simulink library "Enrg_conv_El_to_Mec_zfCetrax"  (R2016a)
settings: Solver=ode1  StartTime=0.0  StopTime=Inf  FixedStep=0.001  RelTol=1e-3
undefined symbols (not defined in the file): drvEmot_RefTqeMOT, FirstDrivenAxle_FirstDrivenAxleNoOfEmot, FirstDrivenAxleNoOfEmot, FMIKit, mec_fRollCoeffOverall, mec_iDiffAxle, mec_massVehicle_kg, mec_rWheelDriven, RefTqeMOT, SecondDrivenAxle_SecondDrivenAxleNoOfEmot, SecondDrivenAxleNoOfEmot
libraries: simulink_extras x3, Enrg_conv_El_to_Mec_zfCetrax x3
(part 2 of 3)

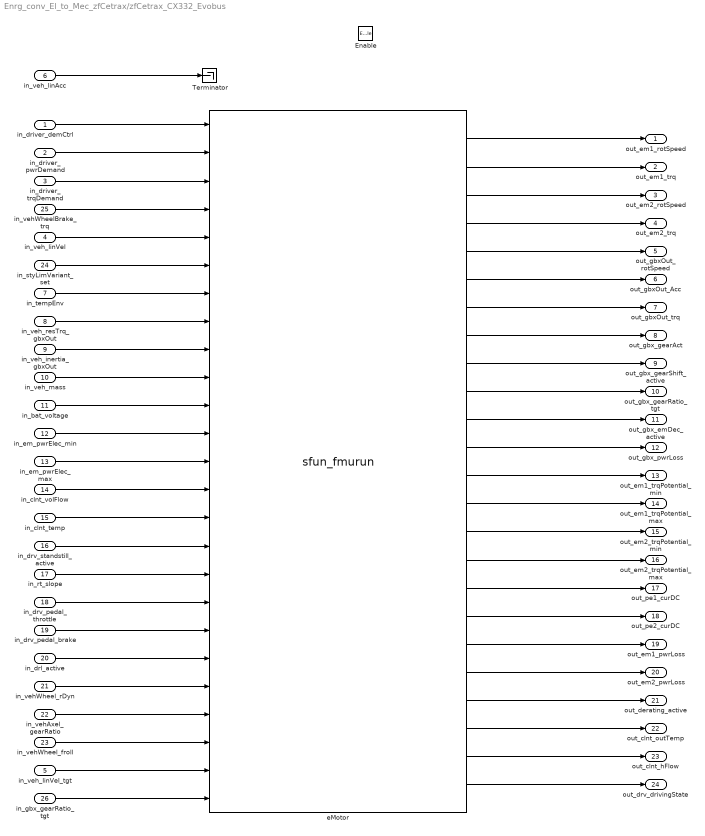
== system Enrg_conv_El_to_Mec_zfCetrax/zfCetrax_CX332_Evobus ==
  in_driver_demCtrl : Inport
  in_driver_pwrDemand : Inport  Port=2
  in_driver_trqDemand : Inport  Port=3
  in_veh_linVel : Inport  Port=4
  in_veh_linVel_tgt : Inport  Port=5
  in_veh_linAcc : Inport  Port=6
  in_tempEnv : Inport  Port=7
  in_veh_resTrq_gbxOut : Inport  Port=8
  in_veh_inertia_gbxOut : Inport  Port=9
  in_veh_mass : Inport  Port=10
  in_bat_voltage : Inport  Port=11
  in_em_pwrElec_min : Inport  Port=12
  in_em_pwrElec_max : Inport  Port=13
  in_clnt_volFlow : Inport  Port=14
  in_clnt_temp : Inport  Port=15
  in_drv_standstill_active : Inport  Port=16
  in_rt_slope : Inport  Port=17
  in_drv_pedal_throttle : Inport  Port=18
  in_drv_pedal_brake : Inport  Port=19
  in_drl_active : Inport  Port=20
  in_vehWheel_rDyn : Inport  Port=21
  in_vehAxel_gearRatio : Inport  Port=22
  in_vehWheel_froll : Inport  Port=23
  in_styLimVariant_set : Inport  Port=24
  in_vehWheelBrake_trq : Inport  Port=25
  in_gbx_gearRatio_tgt : Inport  Port=26
  Enable : EnablePort
  Terminator : Terminator
  eMotor : S-Function  LoadFcn=FMIKit.setSFunctionParameters(gcb)  FunctionName=sfun_fmurun  Parameters='2.0' 1 '{72cfe2f2-dd7d-8c89-a52c-23a74381eb1f}' 'CustomerVar_EvoBusCX332' FMIKit.getUnzipDirectory(gcb) 0 0 0 '' 0 -1 0 0 0 [] [] [] [] char({}) [1 1 1 1 1 1 1 1 1 1 1 1 1 1 1 1 1 1 1 1 1 1 1 1 1] [0 0 0 0 0 0 0 0 0 0 0 0 0 0 0 0 0 0 0 0 0 0 0 0 0] [0 0 0 0 0 0 0 0 0 0 0 0 0 0 0 0 0 0 0 0 0 0 0 0 0] [0 1 2 3 4 5 6 7 8 9 10 11 12 13 14 15 16 17 18 19 20 21 22 23 24] [1 1 1 1 1 1 1 1 1 1 1 1 1 1 1 1 1 1 1 1 1 1 1 1] [0 0 0 0 0 0 0 0 0 0 0 0 0 0 0 0 0 0 0 0 0 0 0 0] [25 26 27 28 29 30 31 32 33 34 35 36 37 38 39 40 41 42 43 44 45 46 47 48]  SFunctionDeploymentMode=off  EnableBusSupport=off
      settings: DeleteFcn=FMIKit.closeBlockDialog(gcbh)  ModelCloseFcn=FMIKit.closeBlockDialog(gcbh)  DestroyFcn=FMIKit.closeBlockDialog(gcbh)  OpenFcn=FMIKit.showBlockDialog(gcbh);  CloseFcn=FMIKit.closeBlockDialog(gcbh)  ParentCloseFcn=FMIKit.closeBlockDialog(gcbh)
      mask Help: eval('FMIKit.showBlockDialogHelp();')
      mask Display:
      | ports = get_param(gcb, 'Ports');
      | 
      | inports = FMIKit.getInportLabels(gcb);
      | 
      | for i = 1:min(numel(inports), ports(1))
      |     port_label('input', i, inports{i})
      | end
      | 
      | outports = FMIKit.getOutportLabels(gcb);
      | 
      | for i = 1:min(numel(outports), ports(2))
      |     port_label('output', i, outports{i})
      | end
      | 
      | if isempty(inports) && isempty(outports)
      |     patch([-20 65, 65 -20], [-20 -20 70 70], [1 1 1])
      |     plot([-2 50 50 -2 -2], [0 0 50 50 0])
      |     patch([-9 12 12 -9 -9], [12 12 20 20 12], [1 1 1])
      |     plot([-9 12 12 -9 -9], [12 12 20 20 12])
      |     patch([-9 12 12 -9 -9], [30 30 38 38 30], [1 1 1])
      |     plot([-9 12 12 -9 -9], [30 30 38 38 30])
      | end
  out_em1_rotSpeed : Outport
  out_em1_trq : Outport  Port=2
  out_em2_rotSpeed : Outport  Port=3
  out_em2_trq : Outport  Port=4
  out_gbxOut_rotSpeed : Outport  Port=5
  out_gbxOut_Acc : Outport  Port=6
  out_gbxOut_trq : Outport  Port=7
  out_gbx_gearAct : Outport  Port=8
  out_gbx_gearShift_active : Outport  Port=9
  out_gbx_gearRatio_tgt : Outport  Port=10
  out_gbx_emDec_active : Outport  Port=11
  out_gbx_pwrLoss : Outport  Port=12
  out_em1_trqPotential_min : Outport  Port=13
  out_em1_trqPotential_max : Outport  Port=14
  out_em2_trqPotential_min : Outport  Port=15
  out_em2_trqPotential_max : Outport  Port=16
  out_pe1_curDC : Outport  Port=17
  out_pe2_curDC : Outport  Port=18
  out_em1_pwrLoss : Outport  Port=19
  out_em2_pwrLoss : Outport  Port=20
  out_derating_active : Outport  Port=21
  out_clnt_outTemp : Outport  Port=22
  out_clnt_hFlow : Outport  Port=23
  out_drv_drivingState : Outport  Port=24
  wires:
  eMotor/24 -> out_drv_drivingState/1
  in_gbx_gearRatio_tgt/1 -> eMotor/25
  in_vehWheel_froll/1 -> eMotor/23
  in_vehAxel_gearRatio/1 -> eMotor/22
  in_vehWheel_rDyn/1 -> eMotor/21
  in_driver_demCtrl/1 -> eMotor/1
  in_driver_trqDemand/1 -> eMotor/3
  in_veh_linVel/1 -> eMotor/5
  in_veh_linVel_tgt/1 -> eMotor/24
  in_tempEnv/1 -> eMotor/7
  in_veh_resTrq_gbxOut/1 -> eMotor/8
  in_veh_inertia_gbxOut/1 -> eMotor/9
  in_veh_mass/1 -> eMotor/10
  in_bat_voltage/1 -> eMotor/11
  in_em_pwrElec_min/1 -> eMotor/12
  in_em_pwrElec_max/1 -> eMotor/13
  in_clnt_volFlow/1 -> eMotor/14
  in_clnt_temp/1 -> eMotor/15
  in_drv_standstill_active/1 -> eMotor/16
  in_rt_slope/1 -> eMotor/17
  in_drv_pedal_throttle/1 -> eMotor/18
  in_drv_pedal_brake/1 -> eMotor/19
  in_drl_active/1 -> eMotor/20
  in_driver_pwrDemand/1 -> eMotor/2
  in_veh_linAcc/1 -> Terminator/1
  eMotor/1 -> out_em1_rotSpeed/1
  eMotor/2 -> out_em1_trq/1
  eMotor/3 -> out_em2_rotSpeed/1
  eMotor/4 -> out_em2_trq/1
  eMotor/5 -> out_gbxOut_rotSpeed/1
  eMotor/6 -> out_gbxOut_Acc/1
  eMotor/7 -> out_gbxOut_trq/1
  eMotor/8 -> out_gbx_gearAct/1
  eMotor/9 -> out_gbx_gearShift_active/1
  eMotor/10 -> out_gbx_gearRatio_tgt/1
  eMotor/11 -> out_gbx_emDec_active/1
  eMotor/12 -> out_gbx_pwrLoss/1
  eMotor/13 -> out_em1_trqPotential_min/1
  eMotor/14 -> out_em1_trqPotential_max/1
  eMotor/15 -> out_em2_trqPotential_min/1
  eMotor/16 -> out_em2_trqPotential_max/1
  eMotor/17 -> out_pe1_curDC/1
  eMotor/18 -> out_pe2_curDC/1
  eMotor/19 -> out_em1_pwrLoss/1
  eMotor/20 -> out_em2_pwrLoss/1
  eMotor/21 -> out_derating_active/1
  eMotor/22 -> out_clnt_outTemp/1
  eMotor/23 -> out_clnt_hFlow/1
  in_styLimVariant_set/1 -> eMotor/6
  in_vehWheelBrake_trq/1 -> eMotor/4

== system Enrg_conv_El_to_Mec_zfCetrax/EDB_DriveEmot_zfCetrax/EMD1_Selection ==
  pti_EMD1_TrqReq_Nm : Inport
  pti_EMD1_ControlMode : Inport  Port=2
  edcu_EMD1_CMD_TorqueRefLim : Inport  Port=3
  edcu_EMD1_CMD_ControlMode : Inport  Port=4
  Bus Creator1 : BusCreator  Inputs=2
  Bus Creator2 : BusCreator  Inputs=2
  Constant2 : Constant  Value=0
  Constant3 : Constant  Value=-1
  Constant4 : Constant  Value=drvEmot_RefTqeMOT
  Logical Operator : Logic  Operator=NOT  AllPortsSameDT=off  OutDataTypeStr=boolean
  Logical Operator1 : Logic  AllPortsSameDT=off  OutDataTypeStr=boolean
  Relational Operator2 : RelationalOperator  Operator===  OutDataTypeStr=boolean
  Relational Operator3 : RelationalOperator  Operator===  OutDataTypeStr=boolean
  Switch : Switch  Criteria=u2 > Threshold
  percent_to_Nm2 : Subsystem
  Signal : Outport
  wires:
  Constant2/1 -> Relational Operator2/2
  Relational Operator2/1 -> Logical Operator1/1
  Constant3/1 -> Relational Operator3/1
  Relational Operator3/1 -> Logical Operator1/2
  edcu_EMD1_CMD_ControlMode/1 -> Bus Creator2/2  "EMD1_ControlMode"
  Switch/1 -> Signal/1
  edcu_EMD1_CMD_TorqueRefLim/1 -> percent_to_Nm2/1(Percentage_Torque)
  Bus Creator2/1 -> Switch/3
  pti_EMD1_ControlMode/1 -> Bus Creator1/2, Relational Operator3/2  "EMD1_ControlMode"
  pti_EMD1_TrqReq_Nm/1 -> Relational Operator2/1, Bus Creator1/1  "EMD1_TrqReq_Nm"
  Constant4/1 -> percent_to_Nm2/2(Reference_Torque)
  percent_to_Nm2/1(Torque_Nm) -> Bus Creator2/1  "EMD1_TrqReq_Nm"
  Logical Operator1/1 -> Logical Operator/1
  Bus Creator1/1 -> Switch/1
  Logical Operator/1 -> Switch/2

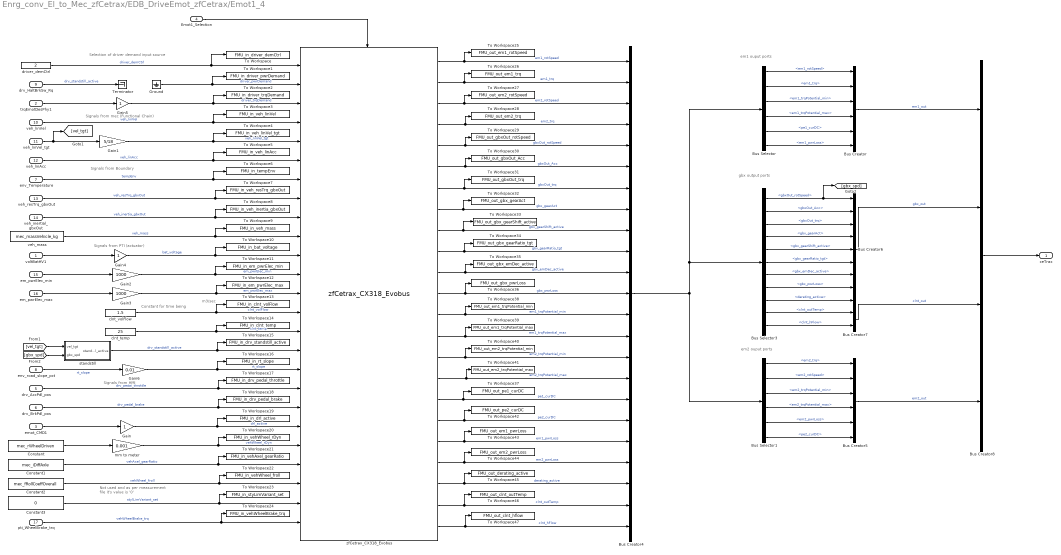
== system Enrg_conv_El_to_Mec_zfCetrax/EDB_DriveEmot_zfCetrax/Emot1_4 ==
  note: em1 ouput ports
  note: Selection of driver demand input source
  note: Signals from Boundary
  note: Signals from HMI
  note: Signals from mec (Functional Chain)
  note: Constant for time being
  note: Signals from PTI (actuator)
  note: em2 ouput ports
  note: gbx output ports
  note: Not used and as per
      | measurement file it's value is '0'
  note: m3/sec
  voltBatHV1 : Inport
  trqEmotDesPhy1 : Inport  Port=2
  emot_CMD1 : Inport  Port=3
  Emot1_Selection : Inport  Port=4
  drv_AccPdl_pos : Inport  Port=5
  drv_BrkPdl_pos : Inport  Port=6
  env_Temperature : Inport  Port=7
  env_road_slope_pct : Inport  Port=8
  drv_HaltBrkSw_Rq : Inport  Port=9
  veh_linVel : Inport  Port=10
  veh_linVel_tgt : Inport  Port=11
  veh_linAcc : Inport  Port=12
  veh_resTrq_gbxOut : Inport  Port=13
  veh_inertial_gbxOut : Inport  Port=14
  em_pwrElec_min : Inport  Port=15
  em_pwrElec_max : Inport  Port=16
  pti_WheelBrake_trq : Inport  Port=17
  Bus Creator : BusCreator  Inputs=6
  Bus Creator4 : BusCreator  Inputs=23
  Bus Creator5 : BusCreator  Inputs=6
  Bus Creator6 : BusCreator  Inputs=9
  Bus Creator7 : BusCreator  Inputs=2
  Bus Creator8 : BusCreator  Inputs=4
  Bus Selector : BusSelector  OutputSignals=em1_rotSpeed,em1_trq,em1_trqPotential_min,em1_trqPotential_max,pe1_curDC,em1_pwrLoss
  Bus Selector1 : BusSelector  OutputSignals=em2_trq,em2_rotSpeed,em2_trqPotential_min,em2_trqPotential_max,em2_pwrLoss,pe2_curDC
  Bus Selector3 : BusSelector  OutputSignals=gbxOut_rotSpeed,gbxOut_Acc,gbxOut_trq,gbx_gearAct,gbx_gearShift_active,gbx_gearRatio_tgt,gbx_emDec_active,gbx_pwrLoss,derating_active,clnt_outTemp,clnt_hFlow
  Constant : Constant  Value=mec_rWheelDriven
  Constant1 : Constant  Value=mec_iDiffAxle
  Constant2 : Constant  Value=mec_fRollCoeffOverall
  Constant3 : Constant  Value=0
  Gain : Gain
  Gain1 : Gain  Gain=5/18
  Gain2 : Gain  Gain=1000
  Gain3 : Gain  Gain=1000
  Gain4 : Gain
  Gain5 : Gain
  Gain6 : Gain  Gain=0.01
  Ground : Ground
  Terminator : Terminator
  To Workspace : ToWorkspace  VariableName=FMU_in_driver_demCtrl  SampleTime=-1
      settings: Save2DSignal=2-D array (concatenate along first dimension)
  To Workspace1 : ToWorkspace  VariableName=FMU_in_driver_pwrDemand  SampleTime=-1
      settings: Save2DSignal=2-D array (concatenate along first dimension)
  To Workspace10 : ToWorkspace  VariableName=FMU_in_bat_voltage  SampleTime=-1
      settings: Save2DSignal=2-D array (concatenate along first dimension)
  To Workspace11 : ToWorkspace  VariableName=FMU_in_em_pwrElec_min  SampleTime=-1
      settings: Save2DSignal=2-D array (concatenate along first dimension)
  To Workspace12 : ToWorkspace  VariableName=FMU_in_em_pwrElec_max  SampleTime=-1
      settings: Save2DSignal=2-D array (concatenate along first dimension)
  To Workspace13 : ToWorkspace  VariableName=FMU_in_clnt_volFlow  SampleTime=-1
      settings: Save2DSignal=2-D array (concatenate along first dimension)
  To Workspace14 : ToWorkspace  VariableName=FMU_in_clnt_temp  SampleTime=-1
      settings: Save2DSignal=2-D array (concatenate along first dimension)
  To Workspace15 : ToWorkspace  VariableName=FMU_in_drv_standstill_active  SampleTime=-1
      settings: Save2DSignal=2-D array (concatenate along first dimension)
  To Workspace16 : ToWorkspace  VariableName=FMU_in_rt_slope  SampleTime=-1
      settings: Save2DSignal=2-D array (concatenate along first dimension)
  To Workspace17 : ToWorkspace  VariableName=FMU_in_drv_pedal_throttle  SampleTime=-1
      settings: Save2DSignal=2-D array (concatenate along first dimension)
  To Workspace18 : ToWorkspace  VariableName=FMU_in_drv_pedal_brake  SampleTime=-1
      settings: Save2DSignal=2-D array (concatenate along first dimension)
  To Workspace19 : ToWorkspace  VariableName=FMU_in_drl_active  SampleTime=-1
      settings: Save2DSignal=2-D array (concatenate along first dimension)
  To Workspace2 : ToWorkspace  VariableName=FMU_in_driver_trqDemand  SampleTime=-1
      settings: Save2DSignal=2-D array (concatenate along first dimension)
  To Workspace20 : ToWorkspace  VariableName=FMU_in_vehWheel_rDyn  SampleTime=-1
      settings: Save2DSignal=2-D array (concatenate along first dimension)
  To Workspace21 : ToWorkspace  VariableName=FMU_in_vehAxel_gearRatio  SampleTime=-1
      settings: Save2DSignal=2-D array (concatenate along first dimension)
  To Workspace22 : ToWorkspace  VariableName=FMU_in_vehWheel_froll  SampleTime=-1
      settings: Save2DSignal=2-D array (concatenate along first dimension)
  To Workspace23 : ToWorkspace  VariableName=FMU_in_styLimVariant_set  SampleTime=-1
      settings: Save2DSignal=2-D array (concatenate along first dimension)
  To Workspace24 : ToWorkspace  VariableName=FMU_in_vehWheelBrake_trq  SampleTime=-1
      settings: Save2DSignal=2-D array (concatenate along first dimension)
  To Workspace25 : ToWorkspace  VariableName=FMU_out_em1_rotSpeed  SampleTime=-1
      settings: Save2DSignal=2-D array (concatenate along first dimension)
  To Workspace26 : ToWorkspace  VariableName=FMU_out_em1_trq  SampleTime=-1
      settings: Save2DSignal=2-D array (concatenate along first dimension)
  To Workspace27 : ToWorkspace  VariableName=FMU_out_em2_rotSpeed  SampleTime=-1
      settings: Save2DSignal=2-D array (concatenate along first dimension)
  To Workspace28 : ToWorkspace  VariableName=FMU_out_em2_trq  SampleTime=-1
      settings: Save2DSignal=2-D array (concatenate along first dimension)
  To Workspace29 : ToWorkspace  VariableName=FMU_out_gbxOut_rotSpeed  SampleTime=-1
      settings: Save2DSignal=2-D array (concatenate along first dimension)
  To Workspace3 : ToWorkspace  VariableName=FMU_in_veh_linVel  SampleTime=-1
      settings: Save2DSignal=2-D array (concatenate along first dimension)
  To Workspace30 : ToWorkspace  VariableName=FMU_out_gbxOut_Acc  SampleTime=-1
      settings: Save2DSignal=2-D array (concatenate along first dimension)
  To Workspace31 : ToWorkspace  VariableName=FMU_out_gbxOut_trq  SampleTime=-1
      settings: Save2DSignal=2-D array (concatenate along first dimension)
  To Workspace32 : ToWorkspace  VariableName=FMU_out_gbx_gearAct  SampleTime=-1
      settings: Save2DSignal=2-D array (concatenate along first dimension)
  To Workspace33 : ToWorkspace  VariableName=FMU_out_gbx_gearShift_active  SampleTime=-1
      settings: Save2DSignal=2-D array (concatenate along first dimension)
  To Workspace34 : ToWorkspace  VariableName=FMU_out_gbx_gearRatio_tgt  SampleTime=-1
      settings: Save2DSignal=2-D array (concatenate along first dimension)
  To Workspace35 : ToWorkspace  VariableName=FMU_out_gbx_emDec_active  SampleTime=-1
      settings: Save2DSignal=2-D array (concatenate along first dimension)
  To Workspace36 : ToWorkspace  VariableName=FMU_out_gbx_pwrLoss  SampleTime=-1
      settings: Save2DSignal=2-D array (concatenate along first dimension)
  To Workspace37 : ToWorkspace  VariableName=FMU_out_pe1_curDC  SampleTime=-1
      settings: Save2DSignal=2-D array (concatenate along first dimension)
  To Workspace38 : ToWorkspace  VariableName=FMU_out_em1_trqPotential_min  SampleTime=-1
      settings: Save2DSignal=2-D array (concatenate along first dimension)
  To Workspace39 : ToWorkspace  VariableName=FMU_out_em1_trqPotential_max  SampleTime=-1
      settings: Save2DSignal=2-D array (concatenate along first dimension)
  To Workspace4 : ToWorkspace  VariableName=FMU_in_veh_linVel_tgt  SampleTime=-1
      settings: Save2DSignal=2-D array (concatenate along first dimension)
  To Workspace40 : ToWorkspace  VariableName=FMU_out_em2_trqPotential_min  SampleTime=-1
      settings: Save2DSignal=2-D array (concatenate along first dimension)
  To Workspace41 : ToWorkspace  VariableName=FMU_out_em2_trqPotential_max  SampleTime=-1
      settings: Save2DSignal=2-D array (concatenate along first dimension)
  To Workspace42 : ToWorkspace  VariableName=FMU_out_pe2_curDC  SampleTime=-1
      settings: Save2DSignal=2-D array (concatenate along first dimension)
  To Workspace43 : ToWorkspace  VariableName=FMU_out_em1_pwrLoss  SampleTime=-1
      settings: Save2DSignal=2-D array (concatenate along first dimension)
  To Workspace44 : ToWorkspace  VariableName=FMU_out_em2_pwrLoss  SampleTime=-1
      settings: Save2DSignal=2-D array (concatenate along first dimension)
  To Workspace45 : ToWorkspace  VariableName=FMU_out_derating_active  SampleTime=-1
      settings: Save2DSignal=2-D array (concatenate along first dimension)
  To Workspace46 : ToWorkspace  VariableName=FMU_out_clnt_outTemp  SampleTime=-1
      settings: Save2DSignal=2-D array (concatenate along first dimension)
  To Workspace47 : ToWorkspace  VariableName=FMU_out_clnt_hflow  SampleTime=-1
      settings: Save2DSignal=2-D array (concatenate along first dimension)
  To Workspace5 : ToWorkspace  VariableName=FMU_in_veh_linAcc  SampleTime=-1
      settings: Save2DSignal=2-D array (concatenate along first dimension)
  To Workspace6 : ToWorkspace  VariableName=FMU_in_tempEnv  SampleTime=-1
      settings: Save2DSignal=2-D array (concatenate along first dimension)
  To Workspace7 : ToWorkspace  VariableName=FMU_in_veh_resTrq_gbxOut  SampleTime=-1
      settings: Save2DSignal=2-D array (concatenate along first dimension)
  To Workspace8 : ToWorkspace  VariableName=FMU_in_veh_inertia_gbxOut  SampleTime=-1
      settings: Save2DSignal=2-D array (concatenate along first dimension)
  To Workspace9 : ToWorkspace  VariableName=FMU_in_veh_mass  SampleTime=-1
      settings: Save2DSignal=2-D array (concatenate along first dimension)
  clnt_temp : Constant  Value=25
  clnt_volFlow : Constant  Value=1.5
  driver_demCtrl : Constant  Value=2
  mm to meter : Gain  Gain=0.001
  standstill : Subsystem
  veh_mass : Constant  Value=mec_massVehicle_kg
  zfCetrax_CX318_Evobus : Enrg_conv_El_to_Mec_zfCetrax/zfCetrax_CX318_Evobus  SystemSampleTime=-1
  ceTrax : Outport
  wires:
  Constant2/1 -> To Workspace22/1, zfCetrax_CX318_Evobus/23  "vehWheel_froll"
  Constant1/1 -> To Workspace21/1, zfCetrax_CX318_Evobus/22  "vehAxel_gearRatio"
  Constant/1 -> mm to meter/1
  emot_CMD1/1 -> Gain/1
  trqEmotDesPhy1/1 -> Gain5/1
  voltBatHV1/1 -> Gain4/1
  Emot1_Selection/1 -> zfCetrax_CX318_Evobus/Enable
  Ground/1 -> To Workspace1/1, zfCetrax_CX318_Evobus/2  "driver_pwrDemand"
  driver_demCtrl/1 -> To Workspace/1, zfCetrax_CX318_Evobus/1  "driver_demCtrl"
  drv_AccPdl_pos/1 -> To Workspace17/1, zfCetrax_CX318_Evobus/18  "drv_pedal_throttle"
  drv_BrkPdl_pos/1 -> To Workspace18/1, zfCetrax_CX318_Evobus/19  "drv_pedal_brake"
  env_Temperature/1 -> To Workspace6/1, zfCetrax_CX318_Evobus/7  "tempEnv"
  env_road_slope_pct/1 -> Gain6/1  "rt_slope"
  veh_mass/1 -> To Workspace9/1, zfCetrax_CX318_Evobus/10  "veh_mass"
  veh_linVel/1 -> To Workspace3/1, zfCetrax_CX318_Evobus/4  "veh_linVel"
  veh_linVel_tgt/1 -> Gain1/1, [vel_tgt]
  veh_linAcc/1 -> To Workspace5/1, zfCetrax_CX318_Evobus/6  "veh_linAcc"
  veh_inertial_gbxOut/1 -> To Workspace8/1, zfCetrax_CX318_Evobus/9  "veh_inertia_gbxOut"
  clnt_temp/1 -> To Workspace14/1, zfCetrax_CX318_Evobus/15  "clnt_temp"
  clnt_volFlow/1 -> To Workspace13/1, zfCetrax_CX318_Evobus/14  "clnt_volFlow"
  em_pwrElec_max/1 -> Gain3/1
  em_pwrElec_min/1 -> Gain2/1
  zfCetrax_CX318_Evobus/8 -> To Workspace32/1, Bus Creator4/8  "gbx_gearAct"
  zfCetrax_CX318_Evobus/10 -> To Workspace34/1, Bus Creator4/10  "gbx_gearRatio_tgt"
  zfCetrax_CX318_Evobus/4 -> To Workspace28/1, Bus Creator4/4  "em2_trq"
  zfCetrax_CX318_Evobus/11 -> To Workspace35/1, Bus Creator4/11  "gbx_emDec_active"
  zfCetrax_CX318_Evobus/12 -> To Workspace36/1, Bus Creator4/12  "gbx_pwrLoss"
  zfCetrax_CX318_Evobus/13 -> To Workspace38/1, Bus Creator4/13  "em1_trqPotential_min"
  zfCetrax_CX318_Evobus/15 -> To Workspace40/1, Bus Creator4/15  "em2_trqPotential_min"
  zfCetrax_CX318_Evobus/9 -> To Workspace33/1, Bus Creator4/9  "gbx_gearShift_active"
  zfCetrax_CX318_Evobus/7 -> To Workspace31/1, Bus Creator4/7  "gbxOut_trq"
  zfCetrax_CX318_Evobus/17 -> Bus Creator4/17, To Workspace37/1  "pe1_curDC"
  zfCetrax_CX318_Evobus/14 -> To Workspace39/1, Bus Creator4/14  "em1_trqPotential_max"
  zfCetrax_CX318_Evobus/1 -> Bus Creator4/1, To Workspace25/1  "em1_rotSpeed"
  zfCetrax_CX318_Evobus/6 -> To Workspace30/1, Bus Creator4/6  "gbxOut_Acc"
  zfCetrax_CX318_Evobus/16 -> To Workspace41/1, Bus Creator4/16  "em2_trqPotential_max"
  zfCetrax_CX318_Evobus/18 -> To Workspace42/1, Bus Creator4/18  "pe2_curDC"
  zfCetrax_CX318_Evobus/2 -> Bus Creator4/2, To Workspace26/1  "em1_trq"
  zfCetrax_CX318_Evobus/3 -> To Workspace27/1, Bus Creator4/3  "em2_rotSpeed"
  zfCetrax_CX318_Evobus/5 -> Bus Creator4/5, To Workspace29/1  "gbxOut_rotSpeed"
  zfCetrax_CX318_Evobus/20 -> To Workspace44/1, Bus Creator4/20  "em2_pwrLoss"
  zfCetrax_CX318_Evobus/19 -> Bus Creator4/19, To Workspace43/1  "em1_pwrLoss"
  zfCetrax_CX318_Evobus/21 -> To Workspace45/1, Bus Creator4/21  "derating_active"
  zfCetrax_CX318_Evobus/23 -> To Workspace47/1, Bus Creator4/23  "clnt_hFlow"
  zfCetrax_CX318_Evobus/22 -> To Workspace46/1, Bus Creator4/22  "clnt_outTemp"
  Bus Creator4/1 -> Bus Selector1/1, Bus Selector3/1, Bus Selector/1
  Gain1/1 -> To Workspace4/1, zfCetrax_CX318_Evobus/5  "veh_linVel_tgt"
  Bus Selector/1 -> Bus Creator/1  "<em1_rotSpeed>"
  Bus Selector/2 -> Bus Creator/2  "<em1_trq>"
  Bus Selector/3 -> Bus Creator/3  "<em1_trqPotential_min>"
  Bus Selector/4 -> Bus Creator/4  "<em1_trqPotential_max>"
  Bus Selector/5 -> Bus Creator/5  "<pe1_curDC>"
  Bus Selector/6 -> Bus Creator/6  "<em1_pwrLoss>"
  Bus Selector1/1 -> Bus Creator5/1  "<em2_trq>"
  Bus Selector1/2 -> Bus Creator5/2  "<em2_rotSpeed>"
  Bus Selector1/3 -> Bus Creator5/3  "<em2_trqPotential_min>"
  Bus Selector1/4 -> Bus Creator5/4  "<em2_trqPotential_max>"
  Bus Selector1/5 -> Bus Creator5/5  "<em2_pwrLoss>"
  Bus Selector1/6 -> Bus Creator5/6  "<pe2_curDC>"
  Bus Selector3/1 -> [gbx_spd], Bus Creator6/1  "<gbxOut_rotSpeed>"
  Bus Selector3/2 -> Bus Creator6/2  "<gbxOut_Acc>"
  Bus Selector3/3 -> Bus Creator6/3  "<gbxOut_trq>"
  Bus Selector3/4 -> Bus Creator6/4  "<gbx_gearAct>"
  Bus Selector3/5 -> Bus Creator6/5  "<gbx_gearShift_active>"
  Bus Selector3/6 -> Bus Creator6/6  "<gbx_gearRatio_tgt>"
  Bus Selector3/7 -> Bus Creator6/7  "<gbx_emDec_active>"
  Bus Selector3/8 -> Bus Creator6/8  "<gbx_pwrLoss>"
  Bus Selector3/9 -> Bus Creator6/9  "<derating_active>"
  Bus Selector3/10 -> Bus Creator7/1  "<clnt_outTemp>"
  Bus Selector3/11 -> Bus Creator7/2  "<clnt_hFlow>"
  Bus Creator/1 -> Bus Creator8/1  "em1_out"
  Bus Creator5/1 -> Bus Creator8/4  "em2_out"
  Bus Creator6/1 -> Bus Creator8/2  "gbx_out"
  Bus Creator7/1 -> Bus Creator8/3  "clnt_out"
  Bus Creator8/1 -> ceTrax/1
  Gain2/1 -> To Workspace11/1, zfCetrax_CX318_Evobus/12  "em_pwrElec_min"
  Gain3/1 -> To Workspace12/1, zfCetrax_CX318_Evobus/13  "em_pwrElec_max"
  mm to meter/1 -> To Workspace20/1, zfCetrax_CX318_Evobus/21  "vehWheel_rDyn"
  Constant3/1 -> To Workspace23/1, zfCetrax_CX318_Evobus/24  "stylLimVariant_set"
  pti_WheelBrake_trq/1 -> To Workspace24/1, zfCetrax_CX318_Evobus/25  "vehWheelBrake_trq"
  standstill/1(standstill_active) -> To Workspace15/1, zfCetrax_CX318_Evobus/16  "drv_standstill_active"
  Gain/1 -> To Workspace19/1, zfCetrax_CX318_Evobus/20  "drl_active"
  Gain4/1 -> To Workspace10/1, zfCetrax_CX318_Evobus/11  "bat_voltage"
  Gain5/1 -> To Workspace2/1, zfCetrax_CX318_Evobus/3  "driver_trqDemand"
  veh_resTrq_gbxOut/1 -> To Workspace7/1, zfCetrax_CX318_Evobus/8  "veh_resTrq_gbxOut"
  Gain6/1 -> To Workspace16/1, zfCetrax_CX318_Evobus/17  "rt_slope"
  drv_HaltBrkSw_Rq/1 -> Terminator/1  "drv_standstill_active"
  [vel_tgt] -> standstill/1(vel_tgt)
  [gbx_spd] -> standstill/2(gbx_spd)

== system Enrg_conv_El_to_Mec_zfCetrax/EDB_DriveEmot_zfCetrax/MotorSelection ==
  MidAxle : Constant  Value=FirstDrivenAxle_FirstDrivenAxleNoOfEmot
  RearAxle : Constant  Value=SecondDrivenAxle_SecondDrivenAxleNoOfEmot
  Truth Table : Truth Table  TreatAsAtomicUnit=on
  Emot1_Selection : Outport
  Emot2_Selection : Outport  Port=2
  Emot3_Selection : Outport  Port=3
  Emot4_Selection : Outport  Port=4
  wires:
  MidAxle/1 -> Truth Table/1(u1)
  RearAxle/1 -> Truth Table/2(u2)
  Truth Table/1(y1) -> Emot1_Selection/1
  Truth Table/2(y2) -> Emot2_Selection/1
  Truth Table/3(y3) -> Emot3_Selection/1
  Truth Table/4(y4) -> Emot4_Selection/1

== system Enrg_conv_El_to_Mec_zfCetrax/EDB_DriveEmot_zfCetrax_CX319/EMD1_Selection ==
  pti_EMD1_TrqReq_Nm : Inport
  pti_EMD1_ControlMode : Inport  Port=2
  edcu_EMD1_CMD_TorqueRefLim : Inport  Port=3
  edcu_EMD1_CMD_ControlMode : Inport  Port=4
  Bus Creator1 : BusCreator  Inputs=2
  Bus Creator2 : BusCreator  Inputs=2
  Constant2 : Constant  Value=0
  Constant3 : Constant  Value=-1
  Constant4 : Constant  Value=RefTqeMOT
  Logical Operator : Logic  Operator=NOT  AllPortsSameDT=off  OutDataTypeStr=boolean
  Logical Operator1 : Logic  AllPortsSameDT=off  OutDataTypeStr=boolean
  Relational Operator2 : RelationalOperator  Operator===  OutDataTypeStr=boolean
  Relational Operator3 : RelationalOperator  Operator===  OutDataTypeStr=boolean
  Switch : Switch  Criteria=u2 > Threshold
  percent_to_Nm2 : Subsystem
  Signal : Outport
  wires:
  Logical Operator/1 -> Switch/2
  Bus Creator1/1 -> Switch/1
  Logical Operator1/1 -> Logical Operator/1
  percent_to_Nm2/1(Torque_Nm) -> Bus Creator2/1  "EMD1_TrqReq_Nm"
  Constant4/1 -> percent_to_Nm2/2(Reference_Torque)
  pti_EMD1_TrqReq_Nm/1 -> Bus Creator1/1, Relational Operator2/1  "EMD1_TrqReq_Nm"
  pti_EMD1_ControlMode/1 -> Relational Operator3/2, Bus Creator1/2  "EMD1_ControlMode"
  Bus Creator2/1 -> Switch/3
  edcu_EMD1_CMD_TorqueRefLim/1 -> percent_to_Nm2/1(Percentage_Torque)
  Switch/1 -> Signal/1
  edcu_EMD1_CMD_ControlMode/1 -> Bus Creator2/2  "EMD1_ControlMode"
  Relational Operator3/1 -> Logical Operator1/2
  Constant3/1 -> Relational Operator3/1
  Relational Operator2/1 -> Logical Operator1/1
  Constant2/1 -> Relational Operator2/2

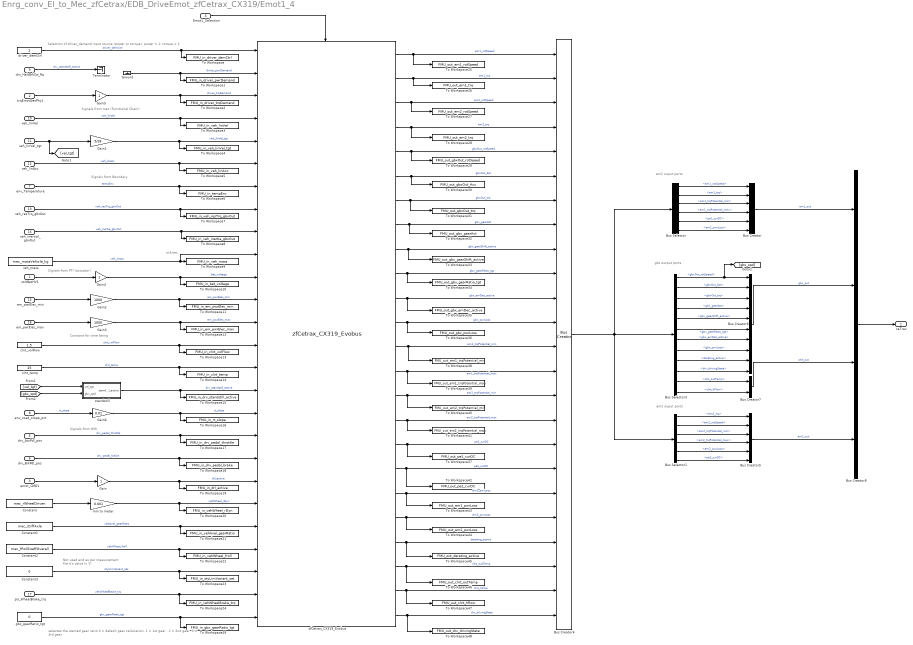
== system Enrg_conv_El_to_Mec_zfCetrax/EDB_DriveEmot_zfCetrax_CX319/Emot1_4 ==
  note: selectes the wanted gear ratio
      | 0 = default gear calculation, 1 = 1st gear , 2 = 2nd gear, 3 = 3rd gear
  note: m3/sec
  note: Not used and as per
      | measurement file it's value is '0'
  note: gbx output ports
  note: em2 ouput ports
  note: Signals from PTI (actuator)
  note: Constant for time being
  note: Signals from mec (Functional Chain)
  note: Signals from HMI
  note: Signals from Boundary
  note: Selection of driver_demand input source (power or torque). power = 1; torque = 2
  note: em1 ouput ports
  voltBatHV1 : Inport
  trqEmotDesPhy1 : Inport  Port=2
  emot_CMD1 : Inport  Port=3
  Emot1_Selection : Inport  Port=4
  drv_AccPdl_pos : Inport  Port=5
  drv_BrkPdl_pos : Inport  Port=6
  env_Temperature : Inport  Port=7
  env_road_slope_pct : Inport  Port=8
  drv_HaltBrkSw_Rq : Inport  Port=9
  veh_linVel : Inport  Port=10
  veh_linVel_tgt : Inport  Port=11
  veh_linAcc : Inport  Port=12
  veh_resTrq_gbxOut : Inport  Port=13
  veh_inertial_gbxOut : Inport  Port=14
  em_pwrElec_min : Inport  Port=15
  em_pwrElec_max : Inport  Port=16
  pti_WheelBrake_trq : Inport  Port=17
  Bus Creator : BusCreator  Inputs=6
  Bus Creator4 : BusCreator  Inputs=24
  Bus Creator5 : BusCreator  Inputs=6
  Bus Creator6 : BusCreator  Inputs=10
  Bus Creator7 : BusCreator  Inputs=2
  Bus Creator8 : BusCreator  Inputs=4
  Bus Selector : BusSelector  OutputSignals=em1_rotSpeed,em1_trq,em1_trqPotential_min,em1_trqPotential_max,pe1_curDC,em1_pwrLoss
  Bus Selector1 : BusSelector  OutputSignals=em2_trq,em2_rotSpeed,em2_trqPotential_min,em2_trqPotential_max,em2_pwrLoss,pe2_curDC
  Bus Selector3 : BusSelector  OutputSignals=gbxOut_rotSpeed,gbxOut_Acc,gbxOut_trq,gbx_gearAct,gbx_gearShift_active,gbx_gearRatio_tgt,gbx_emDec_active,gbx_pwrLoss,derating_active,drv_drivingState,clnt_outTemp,clnt_hFlow
  Constant : Constant  Value=mec_rWheelDriven
  Constant1 : Constant  Value=mec_iDiffAxle
  Constant2 : Constant  Value=mec_fRollCoeffOverall
  Constant3 : Constant  Value=0
  Gain : Gain
  Gain1 : Gain  Gain=5/18
  Gain2 : Gain  Gain=1000
  Gain3 : Gain  Gain=1000
  Gain4 : Gain
  Gain5 : Gain
  Gain6 : Gain  Gain=0.01
  Ground : Ground
  Terminator : Terminator
  To Workspace : ToWorkspace  VariableName=FMU_in_driver_demCtrl  SampleTime=-1
      settings: Save2DSignal=2-D array (concatenate along first dimension)
  To Workspace1 : ToWorkspace  VariableName=FMU_in_driver_pwrDemand  SampleTime=-1
      settings: Save2DSignal=2-D array (concatenate along first dimension)
  To Workspace10 : ToWorkspace  VariableName=FMU_in_bat_voltage  SampleTime=-1
      settings: Save2DSignal=2-D array (concatenate along first dimension)
  To Workspace11 : ToWorkspace  VariableName=FMU_in_em_pwrElec_min  SampleTime=-1
      settings: Save2DSignal=2-D array (concatenate along first dimension)
  To Workspace12 : ToWorkspace  VariableName=FMU_in_em_pwrElec_max  SampleTime=-1
      settings: Save2DSignal=2-D array (concatenate along first dimension)
  To Workspace13 : ToWorkspace  VariableName=FMU_in_clnt_volFlow  SampleTime=-1
      settings: Save2DSignal=2-D array (concatenate along first dimension)
  To Workspace14 : ToWorkspace  VariableName=FMU_in_clnt_temp  SampleTime=-1
      settings: Save2DSignal=2-D array (concatenate along first dimension)
  To Workspace15 : ToWorkspace  VariableName=FMU_in_drv_standstill_active  SampleTime=-1
      settings: Save2DSignal=2-D array (concatenate along first dimension)
  To Workspace16 : ToWorkspace  VariableName=FMU_in_rt_slope  SampleTime=-1
      settings: Save2DSignal=2-D array (concatenate along first dimension)
  To Workspace17 : ToWorkspace  VariableName=FMU_in_drv_pedal_throttle  SampleTime=-1
      settings: Save2DSignal=2-D array (concatenate along first dimension)
  To Workspace18 : ToWorkspace  VariableName=FMU_in_drv_pedal_brake  SampleTime=-1
      settings: Save2DSignal=2-D array (concatenate along first dimension)
  To Workspace19 : ToWorkspace  VariableName=FMU_in_drl_active  SampleTime=-1
      settings: Save2DSignal=2-D array (concatenate along first dimension)
  To Workspace2 : ToWorkspace  VariableName=FMU_in_driver_trqDemand  SampleTime=-1
      settings: Save2DSignal=2-D array (concatenate along first dimension)
  To Workspace20 : ToWorkspace  VariableName=FMU_in_vehWheel_rDyn  SampleTime=-1
      settings: Save2DSignal=2-D array (concatenate along first dimension)
  To Workspace21 : ToWorkspace  VariableName=FMU_in_vehAxel_gearRatio  SampleTime=-1
      settings: Save2DSignal=2-D array (concatenate along first dimension)
  To Workspace22 : ToWorkspace  VariableName=FMU_in_vehWheel_froll  SampleTime=-1
      settings: Save2DSignal=2-D array (concatenate along first dimension)
  To Workspace23 : ToWorkspace  VariableName=FMU_in_styLimVariant_set  SampleTime=-1
      settings: Save2DSignal=2-D array (concatenate along first dimension)
  To Workspace24 : ToWorkspace  VariableName=FMU_in_vehWheelBrake_trq  SampleTime=-1
      settings: Save2DSignal=2-D array (concatenate along first dimension)
  To Workspace25 : ToWorkspace  VariableName=FMU_out_em1_rotSpeed  SampleTime=-1
      settings: Save2DSignal=2-D array (concatenate along first dimension)
  To Workspace26 : ToWorkspace  VariableName=FMU_out_em1_trq  SampleTime=-1
      settings: Save2DSignal=2-D array (concatenate along first dimension)
  To Workspace27 : ToWorkspace  VariableName=FMU_out_em2_rotSpeed  SampleTime=-1
      settings: Save2DSignal=2-D array (concatenate along first dimension)
  To Workspace28 : ToWorkspace  VariableName=FMU_out_em2_trq  SampleTime=-1
      settings: Save2DSignal=2-D array (concatenate along first dimension)
  To Workspace29 : ToWorkspace  VariableName=FMU_out_gbxOut_rotSpeed  SampleTime=-1
      settings: Save2DSignal=2-D array (concatenate along first dimension)
  To Workspace3 : ToWorkspace  VariableName=FMU_in_veh_linVel  SampleTime=-1
      settings: Save2DSignal=2-D array (concatenate along first dimension)
  To Workspace30 : ToWorkspace  VariableName=FMU_out_gbxOut_Acc  SampleTime=-1
      settings: Save2DSignal=2-D array (concatenate along first dimension)
  To Workspace31 : ToWorkspace  VariableName=FMU_out_gbxOut_trq  SampleTime=-1
      settings: Save2DSignal=2-D array (concatenate along first dimension)
  To Workspace32 : ToWorkspace  VariableName=FMU_out_gbx_gearAct  SampleTime=-1
      settings: Save2DSignal=2-D array (concatenate along first dimension)
  To Workspace33 : ToWorkspace  VariableName=FMU_out_gbx_gearShift_active  SampleTime=-1
      settings: Save2DSignal=2-D array (concatenate along first dimension)
  To Workspace34 : ToWorkspace  VariableName=FMU_out_gbx_gearRatio_tgt  SampleTime=-1
      settings: Save2DSignal=2-D array (concatenate along first dimension)
  To Workspace35 : ToWorkspace  VariableName=FMU_out_gbx_emDec_active  SampleTime=-1
      settings: Save2DSignal=2-D array (concatenate along first dimension)
  To Workspace36 : ToWorkspace  VariableName=FMU_out_gbx_pwrLoss  SampleTime=-1
      settings: Save2DSignal=2-D array (concatenate along first dimension)
  To Workspace37 : ToWorkspace  VariableName=FMU_out_pe1_curDC  SampleTime=-1
      settings: Save2DSignal=2-D array (concatenate along first dimension)
  To Workspace38 : ToWorkspace  VariableName=FMU_out_em1_trqPotential_min  SampleTime=-1
      settings: Save2DSignal=2-D array (concatenate along first dimension)
  To Workspace39 : ToWorkspace  VariableName=FMU_out_em1_trqPotential_max  SampleTime=-1
      settings: Save2DSignal=2-D array (concatenate along first dimension)
  To Workspace4 : ToWorkspace  VariableName=FMU_in_veh_linVel_tgt  SampleTime=-1
      settings: Save2DSignal=2-D array (concatenate along first dimension)
  To Workspace40 : ToWorkspace  VariableName=FMU_out_em2_trqPotential_min  SampleTime=-1
      settings: Save2DSignal=2-D array (concatenate along first dimension)
  To Workspace41 : ToWorkspace  VariableName=FMU_out_em2_trqPotential_max  SampleTime=-1
      settings: Save2DSignal=2-D array (concatenate along first dimension)
  To Workspace42 : ToWorkspace  VariableName=FMU_out_pe2_curDC  SampleTime=-1
      settings: Save2DSignal=2-D array (concatenate along first dimension)
  To Workspace43 : ToWorkspace  VariableName=FMU_out_em1_pwrLoss  SampleTime=-1
      settings: Save2DSignal=2-D array (concatenate along first dimension)
  To Workspace44 : ToWorkspace  VariableName=FMU_out_em2_pwrLoss  SampleTime=-1
      settings: Save2DSignal=2-D array (concatenate along first dimension)
  To Workspace45 : ToWorkspace  VariableName=FMU_out_derating_active  SampleTime=-1
      settings: Save2DSignal=2-D array (concatenate along first dimension)
  To Workspace46 : ToWorkspace  VariableName=FMU_out_clnt_outTemp  SampleTime=-1
      settings: Save2DSignal=2-D array (concatenate along first dimension)
  To Workspace47 : ToWorkspace  VariableName=FMU_out_clnt_hflow  SampleTime=-1
      settings: Save2DSignal=2-D array (concatenate along first dimension)
  To Workspace48 : ToWorkspace  VariableName=FMU_out_drv_drivingState  SampleTime=-1
      settings: Save2DSignal=2-D array (concatenate along first dimension)
  To Workspace49 : ToWorkspace  VariableName=FMU_in_gbx_gearRatio_tgt  SampleTime=-1
      settings: Save2DSignal=2-D array (concatenate along first dimension)
  To Workspace5 : ToWorkspace  VariableName=FMU_in_veh_linAcc  SampleTime=-1
      settings: Save2DSignal=2-D array (concatenate along first dimension)
  To Workspace6 : ToWorkspace  VariableName=FMU_in_tempEnv  SampleTime=-1
      settings: Save2DSignal=2-D array (concatenate along first dimension)
  To Workspace7 : ToWorkspace  VariableName=FMU_in_veh_resTrq_gbxOut  SampleTime=-1
      settings: Save2DSignal=2-D array (concatenate along first dimension)
  To Workspace8 : ToWorkspace  VariableName=FMU_in_veh_inertia_gbxOut  SampleTime=-1
      settings: Save2DSignal=2-D array (concatenate along first dimension)
  To Workspace9 : ToWorkspace  VariableName=FMU_in_veh_mass  SampleTime=-1
      settings: Save2DSignal=2-D array (concatenate along first dimension)
  clnt_temp : Constant  Value=25
  clnt_volFlow : Constant  Value=1.5
  driver_demCtrl : Constant  Value=2
  gbx_gearRatio_tgt : Constant  Value=0
  mm to meter : Gain  Gain=0.001
  standstill : Subsystem
  veh_mass : Constant  Value=mec_massVehicle_kg
  zfCetrax_CX319_Evobus : Enrg_conv_El_to_Mec_zfCetrax/zfCetrax_CX319_Evobus  SystemSampleTime=-1
  ceTrax : Outport
  wires:
  Bus Selector3/10 -> Bus Creator6/10  "<drv_drivingState>"
  [gbx_spd] -> standstill/2(gbx_spd)
  [vel_tgt] -> standstill/1(vel_tgt)
  drv_HaltBrkSw_Rq/1 -> Terminator/1  "drv_standstill_active"
  Gain6/1 -> zfCetrax_CX319_Evobus/17, To Workspace16/1  "rt_slope"
  veh_resTrq_gbxOut/1 -> To Workspace7/1, zfCetrax_CX319_Evobus/8  "veh_resTrq_gbxOut"
  Gain5/1 -> zfCetrax_CX319_Evobus/3, To Workspace2/1  "driver_trqDemand"
  Gain4/1 -> zfCetrax_CX319_Evobus/11, To Workspace10/1  "bat_voltage"
  Gain/1 -> To Workspace19/1, zfCetrax_CX319_Evobus/20  "drl_active"
  standstill/1(standstill_active) -> zfCetrax_CX319_Evobus/16, To Workspace15/1  "drv_standstill_active"
  pti_WheelBrake_trq/1 -> zfCetrax_CX319_Evobus/25, To Workspace24/1  "vehWheelBrake_trq"
  Constant3/1 -> zfCetrax_CX319_Evobus/24, To Workspace23/1  "stylLimVariant_set"
  mm to meter/1 -> To Workspace20/1, zfCetrax_CX319_Evobus/21  "vehWheel_rDyn"
  Gain3/1 -> zfCetrax_CX319_Evobus/13, To Workspace12/1  "em_pwrElec_max"
  Gain2/1 -> To Workspace11/1, zfCetrax_CX319_Evobus/12  "em_pwrElec_min"
  Bus Creator8/1 -> ceTrax/1
  Bus Creator7/1 -> Bus Creator8/3  "clnt_out"
  Bus Creator6/1 -> Bus Creator8/2  "gbx_out"
  Bus Creator5/1 -> Bus Creator8/4  "em2_out"
  Bus Creator/1 -> Bus Creator8/1  "em1_out"
  Bus Selector3/12 -> Bus Creator7/2  "<clnt_hFlow>"
  Bus Selector3/11 -> Bus Creator7/1  "<clnt_outTemp>"
  Bus Selector3/9 -> Bus Creator6/9  "<derating_active>"
  Bus Selector3/8 -> Bus Creator6/8  "<gbx_pwrLoss>"
  Bus Selector3/7 -> Bus Creator6/7  "<gbx_emDec_active>"
  Bus Selector3/6 -> Bus Creator6/6  "<gbx_gearRatio_tgt>"
  Bus Selector3/5 -> Bus Creator6/5  "<gbx_gearShift_active>"
  Bus Selector3/4 -> Bus Creator6/4  "<gbx_gearAct>"
  Bus Selector3/3 -> Bus Creator6/3  "<gbxOut_trq>"
  Bus Selector3/2 -> Bus Creator6/2  "<gbxOut_Acc>"
  Bus Selector3/1 -> Bus Creator6/1, [gbx_spd]  "<gbxOut_rotSpeed>"
  Bus Selector1/6 -> Bus Creator5/6  "<pe2_curDC>"
  Bus Selector1/5 -> Bus Creator5/5  "<em2_pwrLoss>"
  Bus Selector1/4 -> Bus Creator5/4  "<em2_trqPotential_max>"
  Bus Selector1/3 -> Bus Creator5/3  "<em2_trqPotential_min>"
  Bus Selector1/2 -> Bus Creator5/2  "<em2_rotSpeed>"
  Bus Selector1/1 -> Bus Creator5/1  "<em2_trq>"
  Bus Selector/6 -> Bus Creator/6  "<em1_pwrLoss>"
  Bus Selector/5 -> Bus Creator/5  "<pe1_curDC>"
  Bus Selector/4 -> Bus Creator/4  "<em1_trqPotential_max>"
  Bus Selector/3 -> Bus Creator/3  "<em1_trqPotential_min>"
  Bus Selector/2 -> Bus Creator/2  "<em1_trq>"
  Bus Selector/1 -> Bus Creator/1  "<em1_rotSpeed>"
  Gain1/1 -> To Workspace4/1, zfCetrax_CX319_Evobus/5  "veh_linVel_tgt"
  Bus Creator4/1 -> Bus Selector/1, Bus Selector3/1, Bus Selector1/1
  zfCetrax_CX319_Evobus/22 -> Bus Creator4/22, To Workspace46/1  "clnt_outTemp"
  zfCetrax_CX319_Evobus/23 -> Bus Creator4/23, To Workspace47/1  "clnt_hFlow"
  zfCetrax_CX319_Evobus/21 -> Bus Creator4/21, To Workspace45/1  "derating_active"
  zfCetrax_CX319_Evobus/19 -> Bus Creator4/19, To Workspace43/1  "em1_pwrLoss"
  zfCetrax_CX319_Evobus/20 -> Bus Creator4/20, To Workspace44/1  "em2_pwrLoss"
  zfCetrax_CX319_Evobus/5 -> Bus Creator4/5, To Workspace29/1  "gbxOut_rotSpeed"
  zfCetrax_CX319_Evobus/3 -> Bus Creator4/3, To Workspace27/1  "em2_rotSpeed"
  zfCetrax_CX319_Evobus/2 -> Bus Creator4/2, To Workspace26/1  "em1_trq"
  zfCetrax_CX319_Evobus/18 -> Bus Creator4/18, To Workspace42/1  "pe2_curDC"
  zfCetrax_CX319_Evobus/16 -> Bus Creator4/16, To Workspace41/1  "em2_trqPotential_max"
  zfCetrax_CX319_Evobus/6 -> Bus Creator4/6, To Workspace30/1  "gbxOut_Acc"
  zfCetrax_CX319_Evobus/1 -> Bus Creator4/1, To Workspace25/1  "em1_rotSpeed"
  zfCetrax_CX319_Evobus/14 -> Bus Creator4/14, To Workspace39/1  "em1_trqPotential_max"
  zfCetrax_CX319_Evobus/17 -> Bus Creator4/17, To Workspace37/1  "pe1_curDC"
  zfCetrax_CX319_Evobus/7 -> Bus Creator4/7, To Workspace31/1  "gbxOut_trq"
  zfCetrax_CX319_Evobus/9 -> Bus Creator4/9, To Workspace33/1  "gbx_gearShift_active"
  zfCetrax_CX319_Evobus/15 -> Bus Creator4/15, To Workspace40/1  "em2_trqPotential_min"
  zfCetrax_CX319_Evobus/13 -> Bus Creator4/13, To Workspace38/1  "em1_trqPotential_min"
  zfCetrax_CX319_Evobus/12 -> Bus Creator4/12, To Workspace36/1  "gbx_pwrLoss"
  zfCetrax_CX319_Evobus/11 -> Bus Creator4/11, To Workspace35/1  "gbx_emDec_active"
  zfCetrax_CX319_Evobus/4 -> Bus Creator4/4, To Workspace28/1  "em2_trq"
  zfCetrax_CX319_Evobus/10 -> Bus Creator4/10, To Workspace34/1  "gbx_gearRatio_tgt"
  zfCetrax_CX319_Evobus/8 -> Bus Creator4/8, To Workspace32/1  "gbx_gearAct"
  em_pwrElec_min/1 -> Gain2/1
  em_pwrElec_max/1 -> Gain3/1
  clnt_volFlow/1 -> zfCetrax_CX319_Evobus/14, To Workspace13/1  "clnt_volFlow"
  clnt_temp/1 -> zfCetrax_CX319_Evobus/15, To Workspace14/1  "clnt_temp"
  veh_inertial_gbxOut/1 -> zfCetrax_CX319_Evobus/9, To Workspace8/1  "veh_inertia_gbxOut"
  veh_linAcc/1 -> zfCetrax_CX319_Evobus/6, To Workspace5/1  "veh_linAcc"
  veh_linVel_tgt/1 -> [vel_tgt], Gain1/1
  veh_linVel/1 -> zfCetrax_CX319_Evobus/4, To Workspace3/1  "veh_linVel"
  veh_mass/1 -> zfCetrax_CX319_Evobus/10, To Workspace9/1  "veh_mass"
  env_road_slope_pct/1 -> Gain6/1  "rt_slope"
  env_Temperature/1 -> To Workspace6/1, zfCetrax_CX319_Evobus/7  "tempEnv"
  drv_BrkPdl_pos/1 -> zfCetrax_CX319_Evobus/19, To Workspace18/1  "drv_pedal_brake"
  drv_AccPdl_pos/1 -> To Workspace17/1, zfCetrax_CX319_Evobus/18  "drv_pedal_throttle"
  driver_demCtrl/1 -> zfCetrax_CX319_Evobus/1, To Workspace/1  "driver_demCtrl"
  Ground/1 -> To Workspace1/1, zfCetrax_CX319_Evobus/2  "driver_pwrDemand"
  Emot1_Selection/1 -> zfCetrax_CX319_Evobus/Enable
  voltBatHV1/1 -> Gain4/1
  trqEmotDesPhy1/1 -> Gain5/1
  emot_CMD1/1 -> Gain/1
  Constant/1 -> mm to meter/1
  Constant1/1 -> To Workspace21/1, zfCetrax_CX319_Evobus/22  "vehAxel_gearRatio"
  Constant2/1 -> zfCetrax_CX319_Evobus/23, To Workspace22/1  "vehWheel_froll"
  gbx_gearRatio_tgt/1 -> zfCetrax_CX319_Evobus/26, To Workspace49/1  "gbx_gearRatio_tgt"
  zfCetrax_CX319_Evobus/24 -> To Workspace48/1, Bus Creator4/24  "drv_drivingState"

== system Enrg_conv_El_to_Mec_zfCetrax/EDB_DriveEmot_zfCetrax_CX319/MotorSelection ==
  MidAxle : Constant  Value=FirstDrivenAxleNoOfEmot
  RearAxle : Constant  Value=SecondDrivenAxleNoOfEmot
  Truth Table : Truth Table  TreatAsAtomicUnit=on
  Emot1_Selection : Outport
  Emot2_Selection : Outport  Port=2
  Emot3_Selection : Outport  Port=3
  Emot4_Selection : Outport  Port=4
  wires:
  Truth Table/4(y4) -> Emot4_Selection/1
  Truth Table/3(y3) -> Emot3_Selection/1
  Truth Table/2(y2) -> Emot2_Selection/1
  Truth Table/1(y1) -> Emot1_Selection/1
  RearAxle/1 -> Truth Table/2(u2)
  MidAxle/1 -> Truth Table/1(u1)

== system Enrg_conv_El_to_Mec_zfCetrax/EDB_DriveEmot_zfCetrax_CX332/EMD1_Selection ==
  pti_EMD1_TrqReq_Nm : Inport
  pti_EMD1_ControlMode : Inport  Port=2
  edcu_EMD1_CMD_TorqueRefLim : Inport  Port=3
  edcu_EMD1_CMD_ControlMode : Inport  Port=4
  Bus Creator1 : BusCreator  Inputs=2
  Bus Creator2 : BusCreator  Inputs=2
  Constant2 : Constant  Value=0
  Constant3 : Constant  Value=-1
  Constant4 : Constant  Value=RefTqeMOT
  Logical Operator : Logic  Operator=NOT  AllPortsSameDT=off  OutDataTypeStr=boolean
  Logical Operator1 : Logic  AllPortsSameDT=off  OutDataTypeStr=boolean
  Relational Operator2 : RelationalOperator  Operator===  OutDataTypeStr=boolean
  Relational Operator3 : RelationalOperator  Operator===  OutDataTypeStr=boolean
  Switch : Switch  Criteria=u2 > Threshold
  percent_to_Nm2 : Subsystem
  Signal : Outport
  wires:
  Constant2/1 -> Relational Operator2/2
  Relational Operator2/1 -> Logical Operator1/1
  Constant3/1 -> Relational Operator3/1
  Relational Operator3/1 -> Logical Operator1/2
  edcu_EMD1_CMD_ControlMode/1 -> Bus Creator2/2  "EMD1_ControlMode"
  Switch/1 -> Signal/1
  edcu_EMD1_CMD_TorqueRefLim/1 -> percent_to_Nm2/1(Percentage_Torque)
  Bus Creator2/1 -> Switch/3
  pti_EMD1_ControlMode/1 -> Bus Creator1/2, Relational Operator3/2  "EMD1_ControlMode"
  pti_EMD1_TrqReq_Nm/1 -> Relational Operator2/1, Bus Creator1/1  "EMD1_TrqReq_Nm"
  Constant4/1 -> percent_to_Nm2/2(Reference_Torque)
  percent_to_Nm2/1(Torque_Nm) -> Bus Creator2/1  "EMD1_TrqReq_Nm"
  Logical Operator1/1 -> Logical Operator/1
  Bus Creator1/1 -> Switch/1
  Logical Operator/1 -> Switch/2
